simulink model "intel_motor_control_rl"  (Simulink 10.3)
settings: Solver=FixedStepDiscrete  StartTime=0.0  StopTime=0.7  FixedStep=62.5e-6 % 16 kHz  RelTol=1e-3  EnableMultiTasking=on
undefined symbols (not defined in the file or in its folder): I_max, Position_PI_Limit
libraries: dspsrcs4 x2, rllib x1
settings Model: Creator=tchau  LastModifiedBy=eee-user8  MultithreadedSim=on
settings Model: SuppressorTable=|
  | <?xml version="1.0" encoding="UTF-8" standalone="yes" ?>
  | <!DOCTYPE boost_serialization>
  | <boost_serialization signature="serialization::archive" version="17">
  | <DiagnosticSuppressor class_id="0" tracking_level="0" version="7">
  | 	<Table class_id="1" tracking_level="0" version="0">
  | 		<count>1</count>
  | 		<bucket_count>8</bucket_count>
  | 		<item_version>0</item_version>
  | 		<item class_id="2" tracking_level="0" version="0">
  | 			<first class_id="3" tracking_level="0" version="7">
  | 				<Source class_id="4" tracking_level="0" version="0">
  | 					<count>1</count>
  | 					<item_version>0</item_version>
  | 					<item>7415:2</item>
  | 				</Source>
  | 			</first>
  | 			<second class_id="5" tracking_level="0" version="7">
  | 				<SuppressedData class_id="6" tracking_level="0" version="0">
  | 					<count>2</count>
  | 					<bucket_count>8</bucket_count>
  | 					<item_version>0</item_version>
  | 					<item class_id="7" tracking_level="0" version="0">
  | 						<first class_id="8" tracking_level="0" version="7">
  | 							<ID>SimulinkFixedPoint:util:Overflowoccurred</ID>
  | 							<Cause>
  | 								<Source>
  | 									<count>0</count>
  | 									<item_version>0</item_version>
  | 								</Source>
  | 							</Cause>
  | 						</first>
  | 						<second class_id="9" tracking_level="0" version="7">
  | 							<Comment></Comment>
  | 							<User></User>
  | 							<LastModified class_id="10" tracking_level="0" version="0">
  | 								<ptime_date class_id="11" tracking_level="0" version="0">
  | 									<date>20160608</date>
  | 								</ptime_date>
  | 								<ptime_time_duration class_id="12" tracking_level="0" version="1">
  | 									<is_special>0</is_special>
  | 									<time_duration_hours>15</time_duration_hours>
  | 									<time_duration_minutes>23</time_duration_minutes>
  | 									<time_duration_seconds>17</time_duration_seconds>
  | 									<time_duration_fractional_seconds>0</time_duration_fractional_seconds>
  | 								</ptime_time_duration>
  | 							</LastModified>
  | 							<SuppressionType>1</SuppressionType>
  | 						</second>
  | 					</item>
  | 					<item>
  | 						<first>
  | 							<ID>Simulink:DataType:WarningOverFlowDetected</ID>
  | 							<Cause>
  | 								<Source>
  | 									<count>0</count>
  | 									<item_version>0</item_version>
  | 								</Source>
  | 							</Cause>
  | 						</first>
  | 						<second>
  | 							<Comment></Comment>
  | 							<User></User>
  | 							<LastModified>
  | 								<ptime_date>
  | 									<date>20160608</date>
  | 								</ptime_date>
  | 								<ptime_time_duration>
  | 									<is_special>0</is_special>
  | 									<time_duration_hours>15</time_duration_hours>
  | 									<time_duration_minutes>23</time_duration_minutes>
  | 									<time_duration_seconds>17</time_duration_seconds>
  | 									<time_duration_fractional_seconds>0</time_duration_fractional_seconds>
  | 								</ptime_time_duration>
  | 							</LastModified>
  | 							<SuppressionType>1</SuppressionType>
  | 						</second>
  | 					</item>
  | 				</SuppressedData>
  | 			</second>
  | 		</item>
  | 	</Table>
  | </DiagnosticSuppressor>
  | 
  | </boost_serialization>
  | 
  | </boost_serialization>
settings DataIOCC: SignalLoggingSaveFormat=Dataset  SaveOutput=off  SignalLogging=off  DSMLogging=off  SaveTime=off
settings OptimizationCC: BlockReduction=off  ConditionallyExecuteInputs=off  DefaultParameterBehavior=Inlined  InlineInvariantSignals=on  ExpressionDepthLimit=128  EfficientFloat2IntCast=on  SimCompilerOptimization=on
settings DebuggingCC: AlgebraicLoopMsg=error  UnderspecifiedInitializationDetection=Simplified  MergeDetectMultiDrivingBlocksExec=error  SolverPrmCheckMsg=warning  SingleTaskRateTransMsg=error  FcnCallInpInsideContextMsg=error  StateNameClashWarn=none
settings HardwareCC: ProdHWDeviceType=ASIC/FPGA->ASIC/FPGA  TargetBitPerPointer=64  TargetBitPerSizeT=64  TargetBitPerPtrDiffT=64  TargetLongLongMode=on  TargetIntDivRoundTo=Zero  TargetEndianess=LittleEndian  TargetWordSize=64  TargetHWDeviceType=MATLAB Host  ProdEqTarget=off
settings GRTTargetCC: CombineOutputUpdateFcns=on  MatFileLogging=off  SupportNonFinite=off  GRTInterface=off

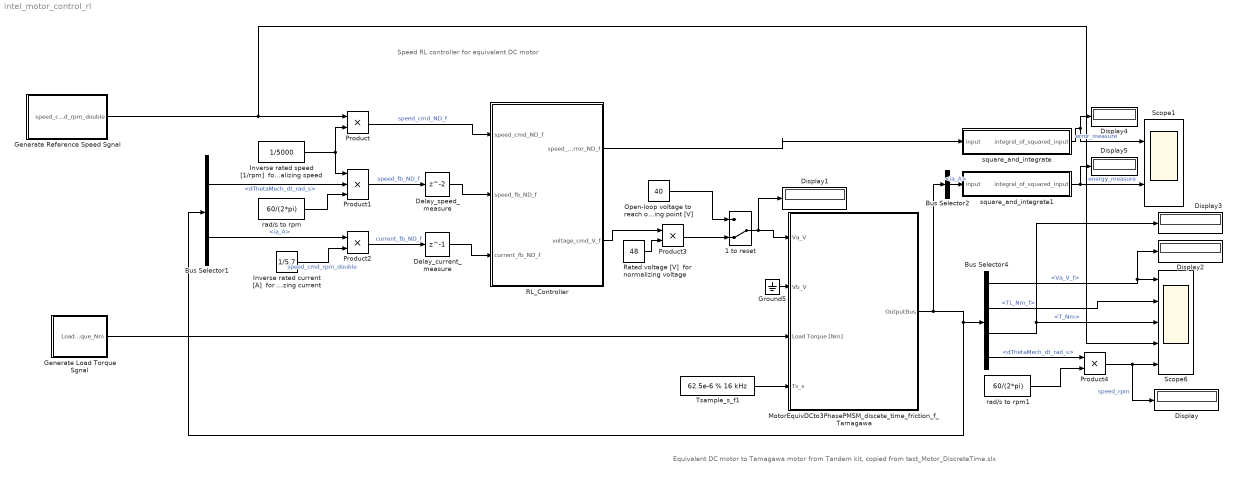
== system intel_motor_control_rl ==
  note: Equivalent DC motor to Tamagawa motor from Tandem kit,
      | copied from test_Motor_DiscreteTime.slx
  note: Speed RL controller
      | for equivalent DC motor
  1 to reset : ManualSwitch  CurrentSetting=0
  Bus Selector1 : BusSelector  OutputSignals=dThetaMech_dt_rad_s,ia_A
  Bus Selector2 : BusSelector  OutputSignals=ia_A
  Bus Selector4 : BusSelector  OutputSignals=Va_V_f,TL_Nm_f,T_Nm,dThetaMech_dt_rad_s
  Delay_current_measure : Delay  DelayLength=1  InitialCondition=0
  Delay_speed_measure : Delay  InitialCondition=0
  Display{,1..5} (6 alike) : Display
  Generate Load Torque Sgnal : Subsystem
  Generate Reference Speed Sgnal : Subsystem
  Ground5 : Ground
  Inverse rated current [A]  for normalizing current : Constant  Value=1/5.7  OutDataTypeStr=double
  Inverse rated speed [1/rpm]  for normalizing speed : Constant  Value=1/5000  OutDataTypeStr=double
  MotorEquivDCto3PhasePMSM_discete_time_friction_f_Tamagawa : Subsystem  mask(Intel PMSM equiv DC){R_ohm=0.68/3, L_H=3e-3/3, Ke_Vs_rad=0.07, Kt_Nm_A=0.07, PolePairs_int=2, J_kgm2=0.165e-4, Tf_Nm=0.02}
      mask prompts: R_ohm "Phase resistance [Ohm]"; L_H "Phase inductance [H]"; Ke_Vs_rad "Back-emf constant kE, based on peak phase values [Vs/rad]"; Kt_Nm_A "Motor torque constant kT, based on peak phase values [Nm/A]"; PolePairs_int "Number of pole pairs (0.5*n poles)  [integer]"; J_kgm2 "Mechanical inertia [kgm^2]"; Tf_Nm "Static friction Tf [Nm]"
      mask help: Intel motor model, equiv DC to PMSM
  Open-loop voltage to  reach operating point [V] : Constant  Value=40  OutDataTypeStr=double
  Product{,2..4} (4 alike) : Product
  Product1 : Product  Inputs=***
  RL_Controller : Subsystem
  Rated voltage [V]  for normalizing voltage : Constant  Value=48  OutDataTypeStr=double
  Scope1 : Scope  NumInputPorts=2
  Scope6 : Scope  NumInputPorts=5
  Tsample_s_f1 : Constant  Value=62.5e-6 % 16 kHz  OutDataTypeStr=double
  rad/s to rpm : Constant  Value=60/(2*pi)  OutDataTypeStr=double
  rad/s to rpm1 : Constant  Value=60/(2*pi)  OutDataTypeStr=double
  square_and_integrate : Subsystem
  square_and_integrate1 : Subsystem
  wires:
  MotorEquivDCto3PhasePMSM_discete_time_friction_f_Tamagawa/1(OutputBus) -> Bus Selector2/1, Bus Selector1/1, Bus Selector4/1
  Bus Selector4/3 -> Scope6/3, Display3/1  "<T_Nm>"
  Ground5/1 -> MotorEquivDCto3PhasePMSM_discete_time_friction_f_Tamagawa/2(Vb_V)
  Bus Selector4/1 -> Display2/1, Scope6/1  "<Va_V_f>"
  Bus Selector4/4 -> Product4/1  "<dThetaMech_dt_rad_s>"
  Product/1 -> RL_Controller/1(speed_cmd_ND_f)  "speed_cmd_ND_f"
  Tsample_s_f1/1 -> MotorEquivDCto3PhasePMSM_discete_time_friction_f_Tamagawa/4(Ts_s)
  Inverse rated speed [1/rpm]  for normalizing speed/1 -> Product1/1, Product/2
  Product1/1 -> Delay_speed_measure/1  "speed_fb_ND_f"
  Bus Selector1/1 -> Product1/2  "<dThetaMech_dt_rad_s>"
  Bus Selector1/2 -> Product2/1  "<ia_A>"
  Inverse rated current [A]  for normalizing current/1 -> Product2/2  "speed_cmd_rpm_double"
  RL_Controller/2(voltage_cmd_V_f) -> Product3/1
  Rated voltage [V]  for normalizing voltage/1 -> Product3/2
  rad/s to rpm/1 -> Product1/3
  Product2/1 -> Delay_current_measure/1  "current_fb_ND_f"
  Product4/1 -> Scope6/5, Display/1  "speed_rpm"
  rad/s to rpm1/1 -> Product4/2
  Open-loop voltage to  reach operating point [V]/1 -> 1 to reset/1
  Product3/1 -> 1 to reset/2
  1 to reset/1 -> Display1/1, MotorEquivDCto3PhasePMSM_discete_time_friction_f_Tamagawa/1(Va_V)
  Bus Selector4/2 -> Scope6/2  "<TL_Nm_f>"
  RL_Controller/1(speed_error_ND_f) -> square_and_integrate/1(input)
  square_and_integrate/1(integral_of_squared_input) -> Scope1/1, Display4/1  "error_measure"
  Bus Selector2/1 -> square_and_integrate1/1(input)  "<ia_A>"
  square_and_integrate1/1(integral_of_squared_input) -> Display5/1, Scope1/2  "energy_measure"
  Delay_speed_measure/1 -> RL_Controller/2(speed_fb_ND_f)
  Delay_current_measure/1 -> RL_Controller/3(current_fb_ND_f)
  Generate Reference Speed Sgnal/1(speed_cmd_rpm_double) -> Scope6/4, Product/1
  Generate Load Torque Sgnal/1(Load_Torque_Nm) -> MotorEquivDCto3PhasePMSM_discete_time_friction_f_Tamagawa/3(Load Torque [Nm])

== system intel_motor_control_rl/Generate Load Torque Sgnal ==
  Product5 : Product
  Random Source1 : dspsrcs4/Random Source  SrcType=Uniform  NormMethod=Ziggurat  CltLength=12  MinVal=-1  MaxVal=1  MeanVal=0  VarVal=1  RepMode=Specify seed  rawSeed=randSeed  IsInherit=off  SampMode=Discrete  SampTime=450*62.5e-6  SampFrame=1  DataType=Double  OutComplex=Real  OutputFrames=off
  Rate Transition1 : RateTransition  OutPortSampleTime=62.5e-6
  Rated torque [Nm] : Constant  Value=0.38  OutDataTypeStr=double
  Load_Torque_Nm : Outport
  wires:
  Product5/1 -> Load_Torque_Nm/1
  Rate Transition1/1 -> Product5/2
  Rated torque [Nm]/1 -> Product5/1
  Random Source1/1 -> Rate Transition1/1

== system intel_motor_control_rl/Generate Reference Speed Sgnal ==
  Random Source : dspsrcs4/Random Source  SrcType=Uniform  NormMethod=Ziggurat  CltLength=12  MinVal=-5000  MaxVal=5000  MeanVal=0  VarVal=1  RepMode=Specify seed  rawSeed=randSeed  IsInherit=off  SampMode=Discrete  SampTime=800*62.5e-6  SampFrame=1  DataType=Double  OutComplex=Real  OutputFrames=off
  Rate Transition : RateTransition  OutPortSampleTime=62.5e-6
  speed_cmd_rpm_double : Outport
  wires:
  Random Source/1 -> Rate Transition/1
  Rate Transition/1 -> speed_cmd_rpm_double/1  "speed_cmd_rpm_double"

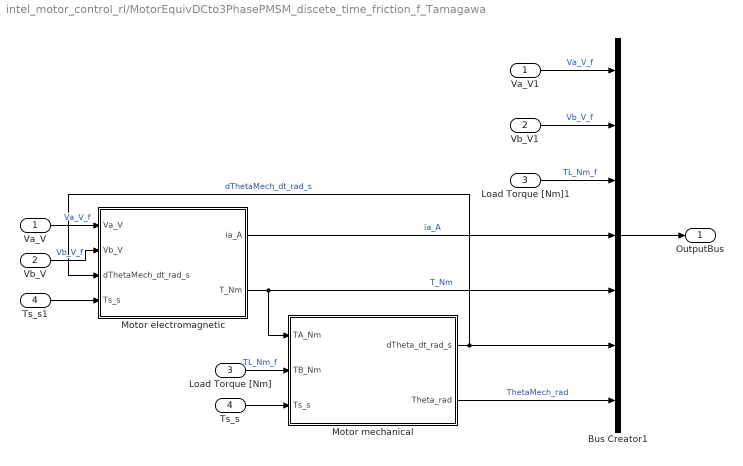
== system intel_motor_control_rl/MotorEquivDCto3PhasePMSM_discete_time_friction_f_Tamagawa ==
  Va_V : Inport
  Vb_V : Inport  Port=2
  Load Torque [Nm] : Inport  Port=3
  Ts_s : Inport  Port=4
  Bus Creator1 : BusCreator  Inputs=7
  Load Torque [Nm]1 : InportShadow  Port=3
  Motor electromagnetic : Subsystem
  Motor mechanical : Subsystem  mask(Inertia){J_kgm2=J_kgm2}
      mask prompts: J_kgm2 "Inertia [kgm^2]"
      mask help:
      | Mechanical inertia with two attachment points A and B.
      | Torque is applied to the inertia from side A and side B.
      | The combined torque acting on the inertia produces acceleration,
      | velocity and displacement. Velocity and displacement are output as these
      | are the states of the system.
  Ts_s1 : InportShadow  Port=4
  Va_V1 : InportShadow
  Vb_V1 : InportShadow  Port=2
  OutputBus : Outport
  wires:
  Ts_s1/1 -> Motor electromagnetic/4(Ts_s)
  Motor mechanical/1(dTheta_dt_rad_s) -> Motor electromagnetic/3(dThetaMech_dt_rad_s), Bus Creator1/6  "dThetaMech_dt_rad_s"
  Ts_s/1 -> Motor mechanical/3(Ts_s)
  Load Torque [Nm]/1 -> Motor mechanical/2(TB_Nm)  "TL_Nm_f"
  Va_V/1 -> Motor electromagnetic/1(Va_V)  "Va_V_f"
  Bus Creator1/1 -> OutputBus/1
  Vb_V/1 -> Motor electromagnetic/2(Vb_V)  "Vb_V_f"
  Va_V1/1 -> Bus Creator1/1  "Va_V_f"
  Vb_V1/1 -> Bus Creator1/2  "Vb_V_f"
  Motor electromagnetic/1(ia_A) -> Bus Creator1/4  "ia_A"
  Motor electromagnetic/2(T_Nm) -> Motor mechanical/1(TA_Nm), Bus Creator1/5  "T_Nm"
  Motor mechanical/2(Theta_rad) -> Bus Creator1/7  "ThetaMech_rad"
  Load Torque [Nm]1/1 -> Bus Creator1/3  "TL_Nm_f"

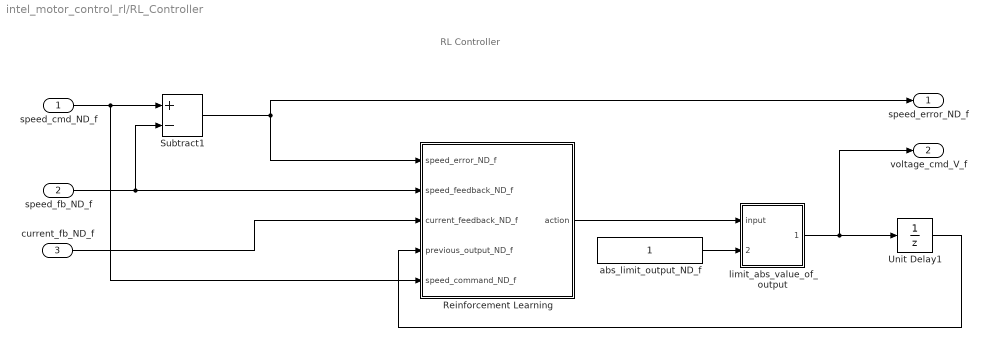
== system intel_motor_control_rl/RL_Controller ==
  note: RL Controller
  speed_cmd_ND_f : Inport
  speed_fb_ND_f : Inport  Port=2  PortDimensions=1
  current_fb_ND_f : Inport  Port=3  PortDimensions=1
  Reinforcement Learning : Subsystem
  Subtract1 : Sum  Inputs=+-
  Unit Delay1 : UnitDelay  SampleTime=-1  HasFrameUpgradeWarning=on
  abs_limit_output_ND_f : Constant  OutDataTypeStr=double
  limit_abs_value_of_output : Subsystem
  speed_error_ND_f : Outport
  voltage_cmd_V_f : Outport  Port=2
  wires:
  limit_abs_value_of_output/1(output) -> voltage_cmd_V_f/1, Unit Delay1/1
  Reinforcement Learning/1(action) -> limit_abs_value_of_output/1(input)
  Unit Delay1/1 -> Reinforcement Learning/4(previous_output_ND_f)
  current_fb_ND_f/1 -> Reinforcement Learning/3(current_feedback_ND_f)
  Subtract1/1 -> speed_error_ND_f/1, Reinforcement Learning/1(speed_error_ND_f)
  speed_fb_ND_f/1 -> Subtract1/2, Reinforcement Learning/2(speed_feedback_ND_f)
  speed_cmd_ND_f/1 -> Reinforcement Learning/5(speed_command_ND_f), Subtract1/1
  abs_limit_output_ND_f/1 -> limit_abs_value_of_output/2(abs_max)

== system intel_motor_control_rl/square_and_integrate ==
  input : Inport
  Add : Sum
  Product6 : Product  Inputs=***
  Tsample_s_f2 : Constant  Value=62.5e-6 % 16 kHz  OutDataTypeStr=double
  delay_to_integrate : Delay  DelayLength=1  InitialCondition=0
  integral_of_squared_input : Outport
  wires:
  delay_to_integrate/1 -> integral_of_squared_input/1, Add/2
  Product6/1 -> Add/1
  Tsample_s_f2/1 -> Product6/3
  Add/1 -> delay_to_integrate/1
  input/1 -> Product6/1, Product6/2

== system intel_motor_control_rl/square_and_integrate1 ==
  input : Inport
  Add : Sum
  Product6 : Product  Inputs=***
  Tsample_s_f2 : Constant  Value=62.5e-6 % 16 kHz  OutDataTypeStr=double
  delay_to_integrate : Delay  DelayLength=1  InitialCondition=0
  integral_of_squared_input : Outport
  wires:
  input/1 -> Product6/2, Product6/1
  Add/1 -> delay_to_integrate/1
  Tsample_s_f2/1 -> Product6/3
  Product6/1 -> Add/1
  delay_to_integrate/1 -> Add/2, integral_of_squared_input/1

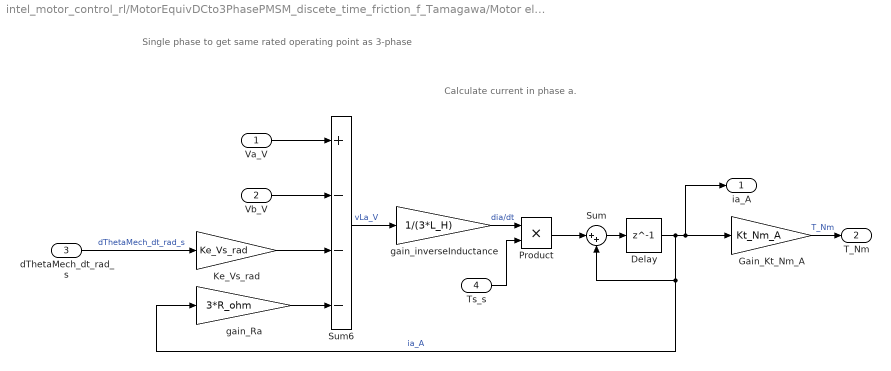
== system intel_motor_control_rl/MotorEquivDCto3PhasePMSM_discete_time_friction_f_Tamagawa/Motor electromagnetic ==
  note: Single phase to get same rated operating point as 3-phase
  note: Calculate current in phase a.
  Va_V : Inport
  Vb_V : Inport  Port=2
  dThetaMech_dt_rad_s : Inport  Port=3
  Ts_s : Inport  Port=4
  Delay : Delay  DelayLength=1
  Gain_Kt_Nm_A : Gain  Gain=Kt_Nm_A
  Ke_Vs_rad : Gain  Gain=Ke_Vs_rad
  Product : Product
  Sum : Sum  Inputs=|++
  Sum6 : Sum  Inputs=+---
  gain_Ra : Gain  Gain=3*R_ohm
  gain_inverseInductance : Gain  Gain=1/(3*L_H)
  ia_A : Outport
  T_Nm : Outport  Port=2
  wires:
  Ts_s/1 -> Product/2
  Sum/1 -> Delay/1
  Product/1 -> Sum/1
  Delay/1 -> gain_Ra/1, Sum/2, Gain_Kt_Nm_A/1, ia_A/1  "ia_A"
  gain_Ra/1 -> Sum6/4
  gain_inverseInductance/1 -> Product/1  "dia/dt"
  Ke_Vs_rad/1 -> Sum6/3
  Sum6/1 -> gain_inverseInductance/1  "vLa_V"
  Vb_V/1 -> Sum6/2
  dThetaMech_dt_rad_s/1 -> Ke_Vs_rad/1  "dThetaMech_dt_rad_s"
  Gain_Kt_Nm_A/1 -> T_Nm/1  "T_Nm"
  Va_V/1 -> Sum6/1

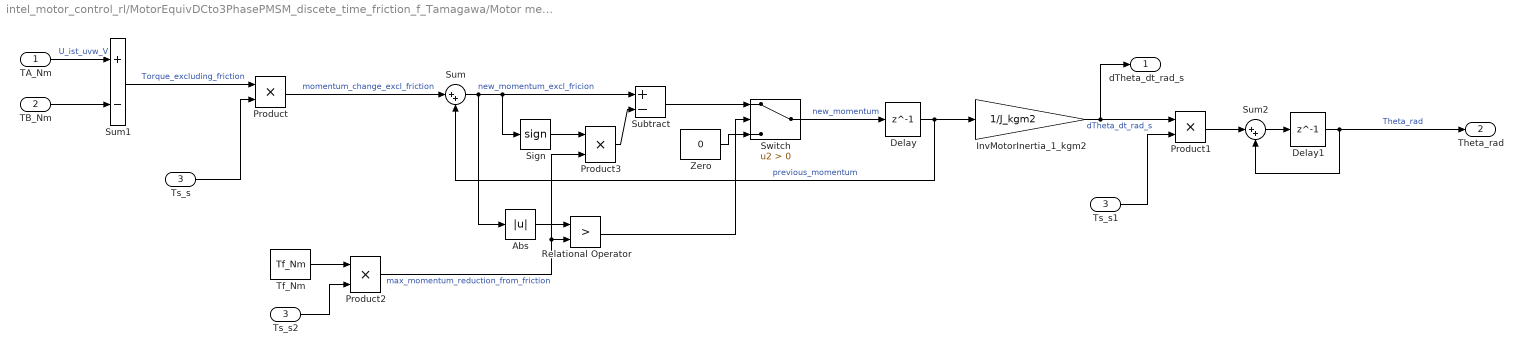
== system intel_motor_control_rl/MotorEquivDCto3PhasePMSM_discete_time_friction_f_Tamagawa/Motor mechanical ==
  TA_Nm : Inport
  TB_Nm : Inport  Port=2
  Ts_s : Inport  Port=3
  Abs : Abs
  Delay : Delay  DelayLength=1
  Delay1 : Delay  DelayLength=1
  InvMotorInertia_1_kgm2 : Gain  Gain=1/J_kgm2
  Product{,1..3} (4 alike) : Product
  Relational Operator : RelationalOperator  Operator=>  OutDataTypeStr=boolean  RndMeth=Nearest
  Sign : Signum
  Subtract : Sum  Inputs=+-
  Sum : Sum  Inputs=|++
  Sum1 : Sum  Inputs=+-
  Sum2 : Sum  Inputs=|++
  Switch : Switch  Criteria=u2 > Threshold
  Tf_Nm : Constant  Value=Tf_Nm
  Ts_s1 : InportShadow  Port=3
  Ts_s2 : InportShadow  Port=3
  Zero : Constant  Value=0
  dTheta_dt_rad_s : Outport
  Theta_rad : Outport  Port=2
  wires:
  Product1/1 -> Sum2/1
  Sum2/1 -> Delay1/1
  Delay1/1 -> Theta_rad/1, Sum2/2  "Theta_rad"
  Sum/1 -> Abs/1, Sign/1, Subtract/1  "new_momentum_excl_fricion"
  Product/1 -> Sum/1  "momentum_change_excl_friction"
  Ts_s/1 -> Product/2
  Sum1/1 -> Product/1  "Torque_excluding_friction"
  TB_Nm/1 -> Sum1/2
  TA_Nm/1 -> Sum1/1  "U_ist_uvw_V"
  Ts_s1/1 -> Product1/2
  Delay/1 -> InvMotorInertia_1_kgm2/1, Sum/2  "previous_momentum"
  Tf_Nm/1 -> Product2/1
  Ts_s2/1 -> Product2/2
  Product2/1 -> Product3/2, Relational Operator/2  "max_momentum_reduction_from_friction"
  Abs/1 -> Relational Operator/1
  Relational Operator/1 -> Switch/2
  Sign/1 -> Product3/1
  Product3/1 -> Subtract/2
  Subtract/1 -> Switch/1
  Zero/1 -> Switch/3
  Switch/1 -> Delay/1  "new_momentum"
  InvMotorInertia_1_kgm2/1 -> dTheta_dt_rad_s/1, Product1/1  "dTheta_dt_rad_s"

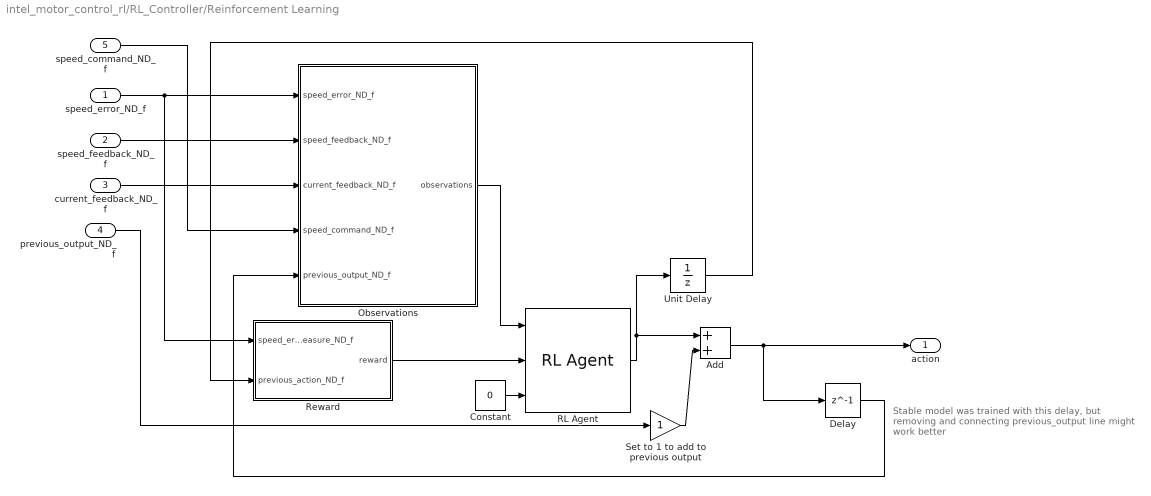
== system intel_motor_control_rl/RL_Controller/Reinforcement Learning ==
  note: Stable model was trained with this delay, but removing and connecting previous_output line might work better
  speed_error_ND_f : Inport
  speed_feedback_ND_f : Inport  Port=2
  current_feedback_ND_f : Inport  Port=3
  previous_output_ND_f : Inport  Port=4
  speed_command_ND_f : Inport  Port=5
  Add : Sum
  Constant : Constant  Value=0
  Delay : Delay  DelayLength=1
  Observations : Subsystem
  RL Agent : rllib/RL Agent  Agent=agent  ExternalActionAsInput=off  ProvideCumRwd=off  TreatAsDirectFeedthrough=on
  Reward : Subsystem
  Set to 1 to add to previous output : Gain
  Unit Delay : UnitDelay  SampleTime=-1  HasFrameUpgradeWarning=on
  action : Outport
  wires:
  Observations/1(observations) -> RL Agent/1
  Reward/1(reward) -> RL Agent/2
  Constant/1 -> RL Agent/3
  speed_error_ND_f/1 -> Observations/1(speed_error_ND_f), Reward/1(speed_error_measure_ND_f)
  speed_feedback_ND_f/1 -> Observations/2(speed_feedback_ND_f)
  current_feedback_ND_f/1 -> Observations/3(current_feedback_ND_f)
  Add/1 -> Delay/1, action/1
  RL Agent/1 -> Add/1, Unit Delay/1
  Delay/1 -> Observations/5(previous_output_ND_f)
  speed_command_ND_f/1 -> Observations/4(speed_command_ND_f)
  Set to 1 to add to previous output/1 -> Add/2
  Unit Delay/1 -> Reward/2(previous_action_ND_f)
  previous_output_ND_f/1 -> Set to 1 to add to previous output/1

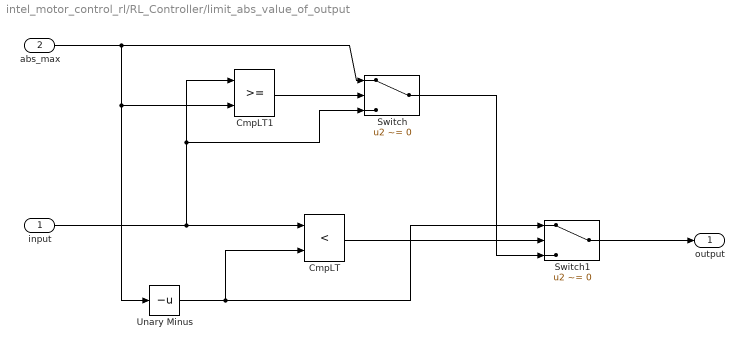
== system intel_motor_control_rl/RL_Controller/limit_abs_value_of_output ==
  input : Inport
  abs_max : Inport  Port=2
  CmpLT : RelationalOperator  Operator=<  OutDataTypeStr=boolean  RndMeth=Nearest
  CmpLT1 : RelationalOperator  OutDataTypeStr=boolean  RndMeth=Nearest
  Switch : Switch  Criteria=u2 ~= 0  Threshold=Position_PI_Limit  ZeroCross=off
  Switch1 : Switch  Criteria=u2 ~= 0  Threshold=I_max  ZeroCross=off
  Unary Minus : UnaryMinus
  output : Outport
  wires:
  Unary Minus/1 -> CmpLT/2, Switch1/1
  Switch1/1 -> output/1
  Switch/1 -> Switch1/3
  CmpLT/1 -> Switch1/2
  input/1 -> CmpLT/1, Switch/3, CmpLT1/1
  abs_max/1 -> Unary Minus/1, CmpLT1/2, Switch/1
  CmpLT1/1 -> Switch/2

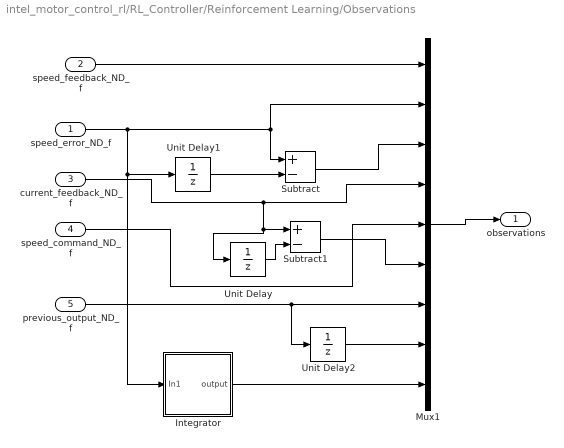
== system intel_motor_control_rl/RL_Controller/Reinforcement Learning/Observations ==
  speed_error_ND_f : Inport
  speed_feedback_ND_f : Inport  Port=2
  current_feedback_ND_f : Inport  Port=3
  speed_command_ND_f : Inport  Port=4
  previous_output_ND_f : Inport  Port=5
  Integrator : Subsystem
  Mux1 : Mux  Inputs=9
  Subtract : Sum  Inputs=+-
  Subtract1 : Sum  Inputs=+-
  Unit Delay : UnitDelay  SampleTime=-1  HasFrameUpgradeWarning=on
  Unit Delay1 : UnitDelay  SampleTime=-1  HasFrameUpgradeWarning=on
  Unit Delay2 : UnitDelay  SampleTime=-1  HasFrameUpgradeWarning=on
  observations : Outport  VectorParamsAs1DForOutWhenUnconnected=off
  wires:
  Mux1/1 -> observations/1
  speed_feedback_ND_f/1 -> Mux1/1
  current_feedback_ND_f/1 -> Subtract1/1, Unit Delay/1, Mux1/4
  Unit Delay1/1 -> Subtract/2
  Subtract/1 -> Mux1/3
  previous_output_ND_f/1 -> Unit Delay2/1, Mux1/7
  speed_command_ND_f/1 -> Mux1/5
  Unit Delay/1 -> Subtract1/2
  Subtract1/1 -> Mux1/6
  Unit Delay2/1 -> Mux1/8
  speed_error_ND_f/1 -> Unit Delay1/1, Integrator/1(In1), Mux1/2, Subtract/1
  Integrator/1(output) -> Mux1/9

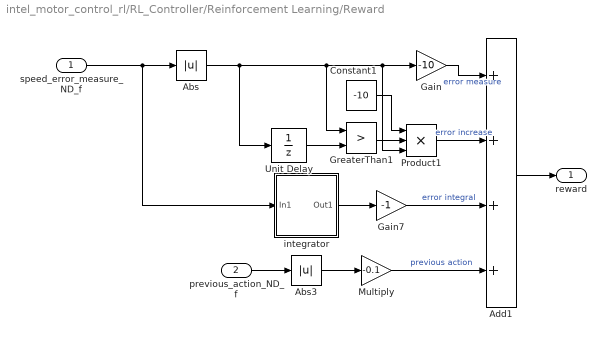
== system intel_motor_control_rl/RL_Controller/Reinforcement Learning/Reward ==
  speed_error_measure_ND_f : Inport
  previous_action_ND_f : Inport  Port=2
  Abs : Abs
  Abs3 : Abs
  Add1 : Sum  Inputs=++++
  Constant1 : Constant  Value=-10
  Gain : Gain  Gain=-10
  Gain7 : Gain  Gain=-1
  GreaterThan1 : RelationalOperator  Operator=>  OutDataTypeStr=boolean  RndMeth=Simplest
  Multiply : Gain  Gain=-0.1
  Product1 : Product  Inputs=3
  Unit Delay : UnitDelay  SampleTime=-1  HasFrameUpgradeWarning=on
  integrator : Subsystem
  reward : Outport  VectorParamsAs1DForOutWhenUnconnected=off
  wires:
  integrator/1(Out1) -> Gain7/1
  GreaterThan1/1 -> Product1/2
  Unit Delay/1 -> GreaterThan1/2
  Multiply/1 -> Add1/4  "previous action"
  Gain7/1 -> Add1/3  "error integral"
  previous_action_ND_f/1 -> Abs3/1
  Abs3/1 -> Multiply/1
  Add1/1 -> reward/1
  Product1/1 -> Add1/2  "error increase"
  Constant1/1 -> Product1/1
  Gain/1 -> Add1/1  "error measure"
  Abs/1 -> Product1/3, Gain/1, GreaterThan1/1, Unit Delay/1
  speed_error_measure_ND_f/1 -> integrator/1(In1), Abs/1

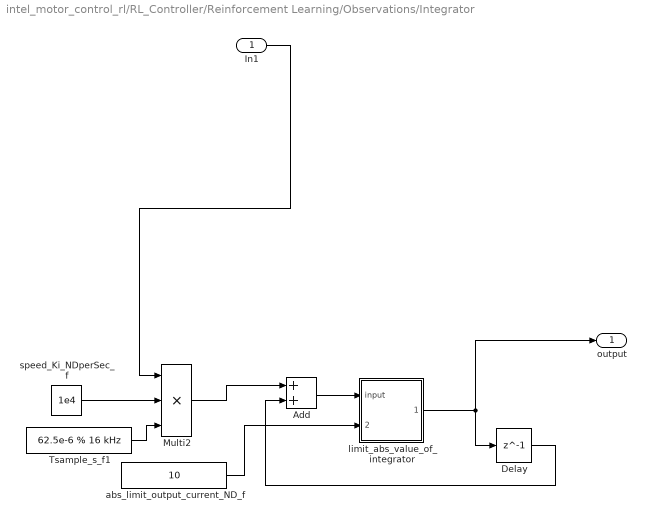
== system intel_motor_control_rl/RL_Controller/Reinforcement Learning/Observations/Integrator ==
  In1 : Inport
  Add : Sum
  Delay : Delay  DelayLength=1  InitialCondition=0
  Multi2 : Product  Inputs=***  RndMeth=Zero  SaturateOnIntegerOverflow=on
  Tsample_s_f1 : Constant  Value=62.5e-6 % 16 kHz  OutDataTypeStr=double
  abs_limit_output_current_ND_f : Constant  Value=10  OutDataTypeStr=double
  limit_abs_value_of_integrator : Subsystem
  speed_Ki_NDperSec_f : Constant  Value=1e4  OutDataTypeStr=double
  output : Outport
  wires:
  Add/1 -> limit_abs_value_of_integrator/1(input)
  Delay/1 -> Add/2
  limit_abs_value_of_integrator/1(output) -> output/1, Delay/1
  abs_limit_output_current_ND_f/1 -> limit_abs_value_of_integrator/2(abs_max)
  Multi2/1 -> Add/1
  In1/1 -> Multi2/1
  Tsample_s_f1/1 -> Multi2/3
  speed_Ki_NDperSec_f/1 -> Multi2/2

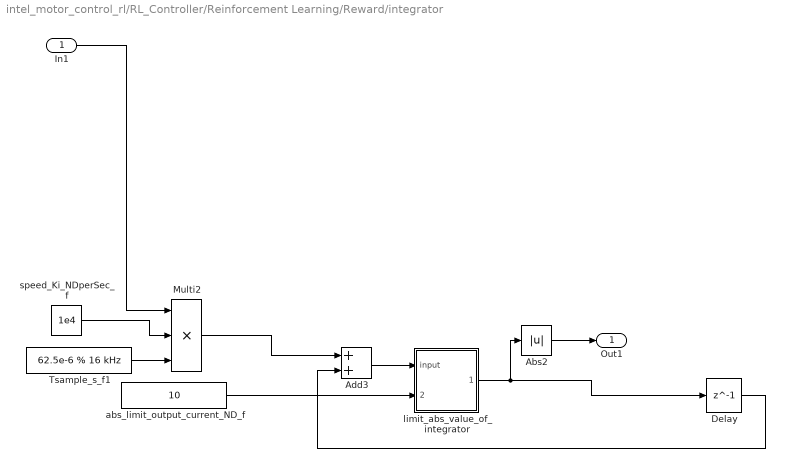
== system intel_motor_control_rl/RL_Controller/Reinforcement Learning/Reward/integrator ==
  In1 : Inport
  Abs2 : Abs
  Add3 : Sum
  Delay : Delay  DelayLength=1  InitialCondition=0
  Multi2 : Product  Inputs=***  RndMeth=Zero  SaturateOnIntegerOverflow=on
  Tsample_s_f1 : Constant  Value=62.5e-6 % 16 kHz  OutDataTypeStr=double
  abs_limit_output_current_ND_f : Constant  Value=10  OutDataTypeStr=double
  limit_abs_value_of_integrator : Subsystem
  speed_Ki_NDperSec_f : Constant  Value=1e4  OutDataTypeStr=double
  Out1 : Outport
  wires:
  abs_limit_output_current_ND_f/1 -> limit_abs_value_of_integrator/2(abs_max)
  limit_abs_value_of_integrator/1(output) -> Abs2/1, Delay/1
  Add3/1 -> limit_abs_value_of_integrator/1(input)
  Abs2/1 -> Out1/1
  In1/1 -> Multi2/1
  Tsample_s_f1/1 -> Multi2/3
  Delay/1 -> Add3/2
  speed_Ki_NDperSec_f/1 -> Multi2/2
  Multi2/1 -> Add3/1

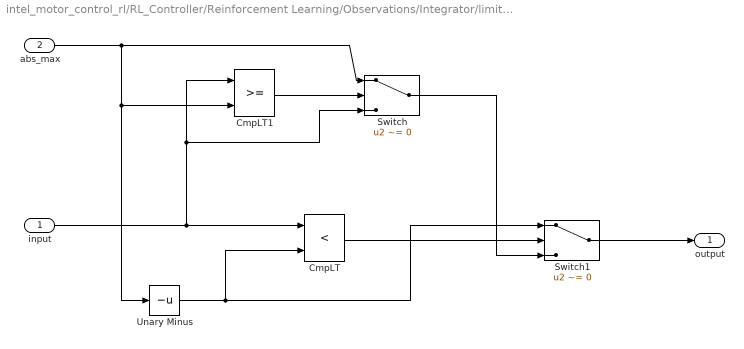
== system intel_motor_control_rl/RL_Controller/Reinforcement Learning/Observations/Integrator/limit_abs_value_of_integrator ==
  input : Inport
  abs_max : Inport  Port=2
  CmpLT : RelationalOperator  Operator=<  OutDataTypeStr=boolean  RndMeth=Nearest
  CmpLT1 : RelationalOperator  OutDataTypeStr=boolean  RndMeth=Nearest
  Switch : Switch  Criteria=u2 ~= 0  Threshold=Position_PI_Limit  ZeroCross=off
  Switch1 : Switch  Criteria=u2 ~= 0  Threshold=I_max  ZeroCross=off
  Unary Minus : UnaryMinus
  output : Outport
  wires:
  CmpLT1/1 -> Switch/2
  abs_max/1 -> Switch/1, CmpLT1/2, Unary Minus/1
  input/1 -> CmpLT1/1, Switch/3, CmpLT/1
  CmpLT/1 -> Switch1/2
  Switch/1 -> Switch1/3
  Switch1/1 -> output/1
  Unary Minus/1 -> Switch1/1, CmpLT/2

== system intel_motor_control_rl/RL_Controller/Reinforcement Learning/Reward/integrator/limit_abs_value_of_integrator ==
  input : Inport
  abs_max : Inport  Port=2
  CmpLT : RelationalOperator  Operator=<  OutDataTypeStr=boolean  RndMeth=Nearest
  CmpLT1 : RelationalOperator  OutDataTypeStr=boolean  RndMeth=Nearest
  Switch : Switch  Criteria=u2 ~= 0  Threshold=Position_PI_Limit  ZeroCross=off
  Switch1 : Switch  Criteria=u2 ~= 0  Threshold=I_max  ZeroCross=off
  Unary Minus : UnaryMinus
  output : Outport
  wires:
  CmpLT1/1 -> Switch/2
  abs_max/1 -> Switch/1, CmpLT1/2, Unary Minus/1
  input/1 -> CmpLT1/1, Switch/3, CmpLT/1
  CmpLT/1 -> Switch1/2
  Switch/1 -> Switch1/3
  Switch1/1 -> output/1
  Unary Minus/1 -> Switch1/1, CmpLT/2
